simulink model "gm_wlanhdlTimeAndFrequencySynchronization"  (R2025a)
settings: Solver=FixedStepDiscrete  StartTime=0.0  StopTime=stopTime  RelTol=1e-3
InitFcn:
  | wlanFrontEndInit;
undefined symbols (not defined in the file or in its folder): a, b, c, Hd, wlanConfig
libraries: simulink x95, hdlsllib x16, hdlmdlgenlib x12, dspsrcs4 x3, dspsigops x3, dsphdlsigops2 x2, dsphdlfiltering2 x2
(part 3 of 11)

== system gm_wlanhdlTimeAndFrequencySynchronization/WLANTimeAndFrequencySynchronization/Coarse Time Sync/Stream Synchronizer ==
  corrValid : Inport  OutDataTypeStr=boolean  PortDimensions=1  SampleTime=5e-08
  dataIn : Inport  Port=2  OutDataTypeStr=fixdt(1, 16, 12)  PortDimensions=1  SampleTime=5e-08
      settings: SignalType=complex
  dataValid : Inport  Port=3  OutDataTypeStr=boolean  PortDimensions=1  SampleTime=5e-08
  Delay1 : RateTransition  InitialCondition=double(0)  OutPortSampleTimeOpt=Multiple of input port sample time  OutPortSampleTimeMultiple=8
  Delay1_absorbed : Delay  DelayLength=0
  Delay{2..4,6} (4 alike) : Delay  DelayLength=double(1)  InitialCondition=0  SampleTime=5e-08
  Delay5 : Delay  DelayLength=double(15)  InitialCondition=0  SampleTime=5e-08
  Logical Operator8 : Logic  Operator=OR  AllPortsSameDT=off  OutDataTypeStr=boolean  SampleTime=6.25e-09
  StreamSyncronizer : Subsystem
  StreamSyncronizer1 : RateTransition  InitialCondition=double(0)  OutPortSampleTimeOpt=Multiple of input port sample time  OutPortSampleTimeMultiple=8
  StreamSyncronizer2 : RateTransition  InitialCondition=double(0)  OutPortSampleTimeOpt=Multiple of input port sample time  OutPortSampleTimeMultiple=8
  crp_out_delay : Delay  DelayLength=double(1)  InitialCondition=0  SampleTime=6.25e-09
  in0_repeat : RateTransition  Integrity=off  Deterministic=off  OutPortSampleTimeOpt=Multiple of input port sample time  OutPortSampleTimeMultiple=1/8
  in1_repeat : RateTransition  Integrity=off  Deterministic=off  OutPortSampleTimeOpt=Multiple of input port sample time  OutPortSampleTimeMultiple=1/8
  in2_repeat : RateTransition  Integrity=off  Deterministic=off  OutPortSampleTimeOpt=Multiple of input port sample time  OutPortSampleTimeMultiple=1/8
  in3_repeat : RateTransition  Integrity=off  Deterministic=off  OutPortSampleTimeOpt=Multiple of input port sample time  OutPortSampleTimeMultiple=1/8
  rd_0 : Delay  DelayLength=double(1)  InitialCondition=0  SampleTime=6.25e-09
  rd_1 : Delay  DelayLength=double(1)  InitialCondition=0  SampleTime=6.25e-09
  dataOut : Outport  SampleTime=5e-08
  validOut : Outport  Port=2  SampleTime=5e-08
  wires:
  Delay3/1 -> validOut/1
  Delay2/1 -> dataOut/1
  StreamSyncronizer/1(dataOut) -> Delay2/1
  StreamSyncronizer2/1 -> StreamSyncronizer/3(push)
  Delay1_absorbed/1 -> StreamSyncronizer/1(pop)
  in1_repeat/1 -> StreamSyncronizer2/1
  in0_repeat/1 -> StreamSyncronizer1/1
  corrValid/1 -> Delay5/1, in3_repeat/1
  rd_1/1 -> Logical Operator8/2
  StreamSyncronizer1/1 -> StreamSyncronizer/2(dataIn)
  crp_out_delay/1 -> Delay1/1
  Delay5/1 -> in2_repeat/1
  Delay1/1 -> Delay1_absorbed/1
  in3_repeat/1 -> rd_1/1
  dataValid/1 -> Delay6/1
  in2_repeat/1 -> rd_0/1
  rd_0/1 -> Logical Operator8/1
  Logical Operator8/1 -> crp_out_delay/1
  StreamSyncronizer/2(validOut) -> Delay3/1
  dataIn/1 -> Delay4/1
  Delay4/1 -> in0_repeat/1
  Delay6/1 -> in1_repeat/1

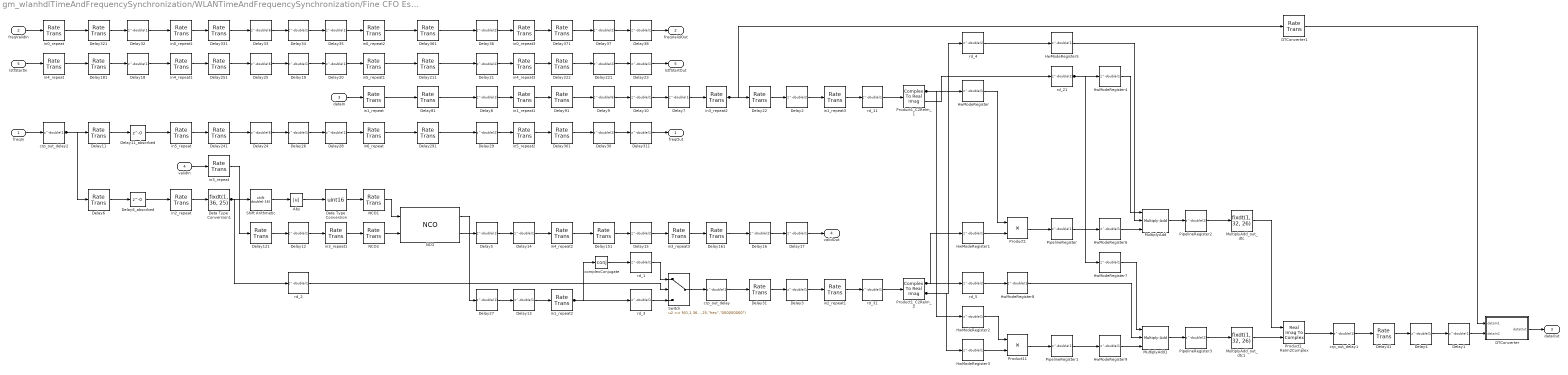
== system gm_wlanhdlTimeAndFrequencySynchronization/WLANTimeAndFrequencySynchronization/Fine CFO Estimation and Correction/Fine CFO Correction ==
  freqIn : Inport  OutDataTypeStr=fixdt(1, 34, 33)  PortDimensions=1  SampleTime=6.25e-09
  freqValidIn : Inport  Port=2  OutDataTypeStr=boolean  PortDimensions=1  SampleTime=5e-08
  dataIn : Inport  Port=3  OutDataTypeStr=fixdt(1, 16, 12)  PortDimensions=1  SampleTime=5e-08
      settings: SignalType=complex
  validIn : Inport  Port=4  OutDataTypeStr=boolean  PortDimensions=1  SampleTime=5e-08
  lstfStartIn : Inport  Port=5  OutDataTypeStr=boolean  PortDimensions=1  SampleTime=5e-08
  Abs : Abs  SampleTime=6.25e-09  OutDataTypeStr=fixdt(1, 36, 25)  SaturateOnIntegerOverflow=off
  DTConverter : Subsystem
  DTConverter1 : RateTransition  InitialCondition=double(0)  OutPortSampleTimeOpt=Multiple of input port sample time  OutPortSampleTimeMultiple=8
  Data Type  Conversion : DataTypeConversion  OutDataTypeStr=uint16  RndMeth=Round  SampleTime=6.25e-09  SaturateOnIntegerOverflow=off
  Data Type  Conversion1 : DataTypeConversion  OutDataTypeStr=fixdt(1, 36, 25)  SampleTime=6.25e-09  SaturateOnIntegerOverflow=off  RndMeth=Floor
  Delay{1,3..5,7..8,10,12..14,17..20,23,26..28,32,34..35,38,311} (23 alike) : Delay  DelayLength=double(1)  InitialCondition=0  SampleTime=5e-08
  Delay{6,11,22,31,41,81,91,121,151,161,181,211,222,241,251,291,301,321,331,361,371} (21 alike) : RateTransition  InitialCondition=double(0)  OutPortSampleTimeOpt=Multiple of input port sample time  OutPortSampleTimeMultiple=8
  Delay11_absorbed : Delay  DelayLength=0
  Delay{2,15..16,21,29..30,36..37,221} (9 alike) : Delay  DelayLength=double(2)  InitialCondition=0  SampleTime=5e-08
  Delay{9,24..25,33} (4 alike) : Delay  DelayLength=double(6)  InitialCondition=0  SampleTime=5e-08
  Delay6_absorbed : Delay  DelayLength=0
  HwModeRegister{,1..9} (10 alike) : Delay  DelayLength=double(1)  InitialCondition=0  SampleTime=6.25e-09
  MultiplyAdd : hdlsllib/HDL Operations/Multiply-Add  Function=c-(a.*b)  datatype=fixdt(1, 33, 26)  DoSatur=off  FMA=off
  MultiplyAdd1 : hdlsllib/HDL Operations/Multiply-Add  Function=c+(a.*b)  datatype=fixdt(1, 33, 26)  DoSatur=off  FMA=off
  MultiplyAdd_out_dtc : DataTypeConversion  OutDataTypeStr=fixdt(1, 32, 26)  SampleTime=6.25e-09  SaturateOnIntegerOverflow=off  RndMeth=Floor
  MultiplyAdd_out_dtc1 : DataTypeConversion  OutDataTypeStr=fixdt(1, 32, 26)  SampleTime=6.25e-09  SaturateOnIntegerOverflow=off  RndMeth=Floor
  NCO : dsphdlsigops2/NCO  PhaseIncrementSource=Input port  PhaseIncrement=100  PhaseOffsetSource=Property  PhaseOffset=0  DitherSource=None  NumDitherBits=4  SamplesPerFrame=1  LUTCompress=off  ResetAction=off  Waveform=Complex exponential  PhasePort=off  SimulateUsing=Code generation  AccumulatorWL=16  PhaseQuantization=on  NumQuantizerAccumulatorBits=16  OutputDataType=Binary point scaling  OutputWL=16  OutputFL=14
  NCO1 : RateTransition  InitialCondition=double(0)  OutPortSampleTimeOpt=Multiple of input port sample time  OutPortSampleTimeMultiple=8
  NCO2 : RateTransition  InitialCondition=double(0)  OutPortSampleTimeOpt=Multiple of input port sample time  OutPortSampleTimeMultiple=8
  PipelineRegister : Delay  DelayLength=double(1)  InitialCondition=0  SampleTime=6.25e-09
  PipelineRegister1 : Delay  DelayLength=double(1)  InitialCondition=0  SampleTime=6.25e-09
  PipelineRegister2 : Delay  DelayLength=double(2)  InitialCondition=0  SampleTime=6.25e-09
  PipelineRegister3 : Delay  DelayLength=double(2)  InitialCondition=0  SampleTime=6.25e-09
  Product1 : Product  Inputs=**  OutDataTypeStr=fixdt(1, 32, 26)  SampleTime=6.25e-09
  Product11 : Product  Inputs=**  OutDataTypeStr=fixdt(1, 32, 26)  SampleTime=6.25e-09
  Product1_C2ReIm_1 : ComplexToRealImag  SampleTime=6.25e-09
  Product1_C2ReIm_2 : ComplexToRealImag  SampleTime=6.25e-09
  Product1_ReIm2Complex : RealImagToComplex  SampleTime=6.25e-09
  Shift Arithmetic : ArithShift  BitShiftNumber=double(-16)  BinPtShiftNumber=double(0)
  Switch : Switch  Threshold="fi(0,1,36,25,\"hex\",\"000000000\")"  OutDataTypeStr=fixdt(1, 16, 14)  SampleTime=6.25e-09  SaturateOnIntegerOverflow=off  InputSameDT=off
  complexConjugate : Math  Operator=conj  SignedPower=on  OutDataTypeStr=fixdt(1, 16, 14)
  crp_out_delay : Delay  DelayLength=double(1)  InitialCondition=0  SampleTime=6.25e-09
  crp_out_delay1 : Delay  DelayLength=double(1)  InitialCondition=0  SampleTime=6.25e-09
  crp_out_delay2 : Delay  DelayLength=double(1)  InitialCondition=0  SampleTime=6.25e-09
  in0_repeat{,1..3} (4 alike) : RateTransition  Integrity=off  Deterministic=off  OutPortSampleTimeOpt=Multiple of input port sample time  OutPortSampleTimeMultiple=1/8
  in1_repeat{,1..3} (4 alike) : RateTransition  Integrity=off  Deterministic=off  OutPortSampleTimeOpt=Multiple of input port sample time  OutPortSampleTimeMultiple=1/8
  in2_repeat : RateTransition  Integrity=off  Deterministic=off  OutPortSampleTimeOpt=Multiple of input port sample time  OutPortSampleTimeMultiple=1/8
  in2_repeat1 : RateTransition  Integrity=off  Deterministic=off  OutPortSampleTimeOpt=Multiple of input port sample time  OutPortSampleTimeMultiple=1/8
  in3_repeat{,1..3} (4 alike) : RateTransition  Integrity=off  Deterministic=off  OutPortSampleTimeOpt=Multiple of input port sample time  OutPortSampleTimeMultiple=1/8
  in4_repeat{,1..3} (4 alike) : RateTransition  Integrity=off  Deterministic=off  OutPortSampleTimeOpt=Multiple of input port sample time  OutPortSampleTimeMultiple=1/8
  in5_repeat : RateTransition  Integrity=off  Deterministic=off  OutPortSampleTimeOpt=Multiple of input port sample time  OutPortSampleTimeMultiple=1/8
  in5_repeat1 : RateTransition  Integrity=off  Deterministic=off  OutPortSampleTimeOpt=Multiple of input port sample time  OutPortSampleTimeMultiple=1/8
  in5_repeat2 : RateTransition  Integrity=off  Deterministic=off  OutPortSampleTimeOpt=Multiple of input port sample time  OutPortSampleTimeMultiple=1/8
  in6_repeat : RateTransition  Integrity=off  Deterministic=off  OutPortSampleTimeOpt=Multiple of input port sample time  OutPortSampleTimeMultiple=1/8
  rd_{1..3,11,31} (5 alike) : Delay  DelayLength=double(1)  InitialCondition=0  SampleTime=6.25e-09
  rd_21 : Delay  DelayLength=double(2)  InitialCondition=0  SampleTime=6.25e-09
  rd_4 : Delay  DelayLength=double(2)  InitialCondition=0  SampleTime=6.25e-09
  rd_5 : Delay  DelayLength=double(2)  InitialCondition=0  SampleTime=6.25e-09
  freqOut : Outport  SampleTime=5e-08  VectorParamsAs1DForOutWhenUnconnected=off
  freqValidOut : Outport  Port=2  SampleTime=5e-08  VectorParamsAs1DForOutWhenUnconnected=off
  dataOut : Outport  Port=3  SampleTime=5e-08  VectorParamsAs1DForOutWhenUnconnected=off
  validOut : Outport  Port=4  SampleTime=5e-08  VectorParamsAs1DForOutWhenUnconnected=off
  lstfStartOut : Outport  Port=5  SampleTime=5e-08  VectorParamsAs1DForOutWhenUnconnected=off
  wires:
  DTConverter/1(dataOut) -> dataOut/1
  Delay4/1 -> Delay1/1
  crp_out_delay1/1 -> Delay41/1
  DTConverter1/1 -> DTConverter/1(dataIn1)
  rd_4/1 -> HwModeRegister5/1
  dataIn/1 -> in1_repeat/1
  Delay29/1 -> in5_repeat2/1
  Delay36/1 -> in0_repeat3/1
  in3_repeat3/1 -> Delay161/1
  NCO/1 -> Delay27/1
  Delay15/1 -> in3_repeat3/1
  NCO/2 -> Delay5/1
  Delay211/1 -> Delay21/1
  in6_repeat/1 -> Delay291/1
  in1_repeat/1 -> Delay81/1
  in5_repeat1/1 -> Delay211/1
  in2_repeat/1 -> Data Type  Conversion1/1
  Delay7/1 -> in3_repeat2/1
  in0_repeat2/1 -> Delay361/1
  in3_repeat1/1 -> NCO2/1
  Data Type  Conversion/1 -> NCO1/1
  Delay35/1 -> in0_repeat2/1
  Delay321/1 -> Delay32/1
  Abs/1 -> Data Type  Conversion/1
  Delay32/1 -> in0_repeat1/1
  Delay19/1 -> Delay20/1
  in0_repeat/1 -> Delay321/1
  Delay151/1 -> Delay15/1
  Delay11_absorbed/1 -> in5_repeat/1
  Shift Arithmetic/1 -> Abs/1
  MultiplyAdd_out_dtc1/1 -> Product1_ReIm2Complex/2
  Delay6/1 -> Delay6_absorbed/1
  Delay11/1 -> Delay11_absorbed/1
  in4_repeat/1 -> Delay181/1
  Delay3/1 -> in2_repeat1/1
  freqValidIn/1 -> in0_repeat/1
  rd_2/1 -> Switch/2
  in1_repeat1/1 -> Delay91/1
  Delay251/1 -> Delay25/1
  Delay26/1 -> Delay28/1
  Delay2/1 -> in1_repeat3/1
  crp_out_delay2/1 -> Delay11/1, Delay6/1
  Delay24/1 -> Delay26/1
  HwModeRegister9/1 -> MultiplyAdd1/3
  Delay25/1 -> Delay19/1
  Delay34/1 -> Delay35/1
  Product1_C2ReIm_2/2 -> HwModeRegister3/1, rd_4/1
  Delay241/1 -> Delay24/1
  Data Type  Conversion1/1 -> Shift Arithmetic/1, rd_2/1
  rd_1/1 -> Switch/1
  Delay181/1 -> Delay18/1
  Product1/1 -> PipelineRegister/1
  Delay6_absorbed/1 -> in2_repeat/1
  PipelineRegister/1 -> HwModeRegister6/1
  Delay1/1 -> DTConverter/2(dataIn2)
  MultiplyAdd1/1 -> PipelineRegister3/1
  PipelineRegister3/1 -> MultiplyAdd_out_dtc1/1
  in0_repeat1/1 -> Delay331/1
  NCO2/1 -> NCO/2
  in4_repeat3/1 -> Delay222/1
  in4_repeat1/1 -> Delay251/1
  freqIn/1 -> crp_out_delay2/1
  Delay5/1 -> Delay14/1
  Delay33/1 -> Delay34/1
  Delay331/1 -> Delay33/1
  HwModeRegister3/1 -> Product11/2
  Delay18/1 -> in4_repeat1/1
  in3_repeat/1 -> Delay121/1
  rd_11/1 -> Product1_C2ReIm_1/1
  validIn/1 -> in3_repeat/1
  Delay28/1 -> in6_repeat/1
  Delay20/1 -> in5_repeat1/1
  Product1_ReIm2Complex/1 -> crp_out_delay1/1
  Delay371/1 -> Delay37/1
  Delay27/1 -> Delay13/1
  Delay121/1 -> Delay12/1
  in5_repeat2/1 -> Delay301/1
  Delay14/1 -> in4_repeat2/1
  PipelineRegister1/1 -> HwModeRegister9/1
  Delay13/1 -> in1_repeat2/1
  Delay361/1 -> Delay36/1
  complexConjugate/1 -> rd_1/1
  Delay222/1 -> Delay221/1
  Delay91/1 -> Delay9/1
  Delay301/1 -> Delay30/1
  in4_repeat2/1 -> Delay151/1
  Delay8/1 -> in1_repeat1/1
  Delay37/1 -> Delay38/1
  Delay21/1 -> in4_repeat3/1
  Delay221/1 -> Delay23/1
  Delay161/1 -> Delay16/1
  HwModeRegister7/1 -> MultiplyAdd1/1
  Delay9/1 -> Delay10/1
  in5_repeat/1 -> Delay241/1
  Delay30/1 -> Delay311/1
  Product1_C2ReIm_1/1 -> HwModeRegister2/1, HwModeRegister/1
  Delay38/1 -> freqValidOut/1
  Delay23/1 -> lstfStartOut/1
  Delay10/1 -> Delay7/1
  Delay311/1 -> freqOut/1
  rd_3/1 -> Switch/3
  Switch/1 -> crp_out_delay/1
  in1_repeat2/1 -> complexConjugate/1, rd_3/1
  HwModeRegister5/1 -> MultiplyAdd/2
  lstfStartIn/1 -> in4_repeat/1
  in3_repeat2/1 -> Delay22/1, DTConverter1/1
  Product1_C2ReIm_1/2 -> rd_21/1
  crp_out_delay/1 -> Delay31/1
  Delay22/1 -> Delay2/1
  Delay16/1 -> Delay17/1
  Delay31/1 -> Delay3/1
  Delay17/1 -> validOut/1
  rd_31/1 -> Product1_C2ReIm_2/1
  in0_repeat3/1 -> Delay371/1
  in1_repeat3/1 -> rd_11/1
  in2_repeat1/1 -> rd_31/1
  HwModeRegister2/1 -> Product11/1
  MultiplyAdd/1 -> PipelineRegister2/1
  Delay81/1 -> Delay8/1
  HwModeRegister/1 -> Product1/1
  NCO1/1 -> NCO/1
  Delay12/1 -> in3_repeat1/1
  PipelineRegister2/1 -> MultiplyAdd_out_dtc/1
  HwModeRegister1/1 -> Product1/2
  Product11/1 -> PipelineRegister1/1
  Product1_C2ReIm_2/1 -> HwModeRegister1/1, rd_5/1
  rd_5/1 -> HwModeRegister8/1
  HwModeRegister8/1 -> MultiplyAdd1/2
  rd_21/1 -> HwModeRegister7/1, HwModeRegister4/1
  Delay291/1 -> Delay29/1
  HwModeRegister4/1 -> MultiplyAdd/1
  HwModeRegister6/1 -> MultiplyAdd/3
  Delay41/1 -> Delay4/1
  MultiplyAdd_out_dtc/1 -> Product1_ReIm2Complex/1
